simulink model "Tools"  (R2022b)
settings: Solver=ode45  StartTime=0.0  StopTime=10.0  RelTol=1e-3  EnableMultiTasking=on
undefined symbols (not defined in the file): AAopti, Copti, gam, nv_remp, Pamb, PRcrit, Rair, table_rdt_AA, Tamb, vect_delta_AA
settings Model: Creator=Boanali  LastModifiedBy=Boanali
settings DataIOCC: LimitDataPoints=on  SaveFormat=Array  SignalLoggingSaveFormat=ModelDataLogs  ReturnWorkspaceOutputs=off  SignalLoggingName=sigsOut
settings OptimizationCC: ReuseModelBlockBuffer=on
settings DebuggingCC: SaveWithParameterizedLinksMsg=none  UnderspecifiedInitializationDetection=Classic  MergeDetectMultiDrivingBlocksExec=none  SignalResolutionControl=TryResolveAllWithWarning  MultiTaskDSMMsg=warning  MultiTaskCondExecSysMsg=none  UnconnectedInputMsg=warning  UnconnectedOutputMsg=warning  UnconnectedLineMsg=warning
settings HardwareCC: ProdBitPerPointer=32  ProdBitPerSizeT=32  ProdBitPerPtrDiffT=32  ProdLargestAtomicFloat=None  ProdIntDivRoundTo=Undefined  ProdEndianess=Unspecified  ProdWordSize=32  ProdHWDeviceType=32-bit Generic  TargetUnknown=on
settings ModelReferenceCC: PropagateSignalLabelsOutOfModel=off
settings GRTTargetCC: CombineOutputUpdateFcns=off  GRTInterface=on
settings ConfigComp: CovMetricSettings=dw  CovSaveCumulativeToWorkspaceVar=on  CovSaveSingleToWorkspaceVar=on

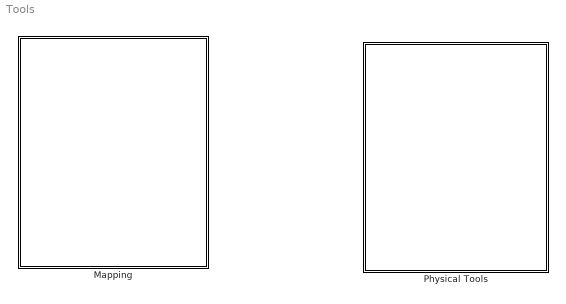
== system Tools ==
  Mapping : Subsystem
      mask Display: disp('CARTOGRAPHIES')
  Physical Tools : Subsystem
      mask Display: disp('PHYSICAL TOOLS')

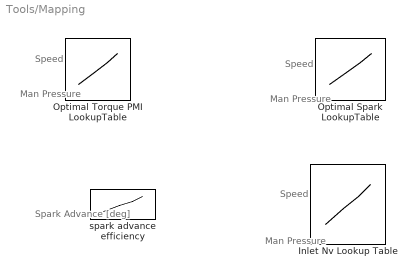
== system Tools/Mapping ==
  note: Speed
  note: Speed
  note: Spark Advance
      | [deg]
  note: Man Pressure
  note: Man Pressure
  note: Speed
  note: Man Pressure
  Inlet Nv Lookup Table : Lookup2D  RowIndex=Ne_remp  ColumnIndex=Pcol_remp  Table=nv_remp
  Optimal Spark LookupTable : Lookup2D  RowIndex=Ne_remp  ColumnIndex=Pcol_remp  Table=AAopti
  Optimal Torque PMI LookupTable : Lookup2D  RowIndex=Ne_remp  ColumnIndex=Pcol_remp  Table=Copti
  spark advance efficiency : Lookup  InputValues=vect_delta_AA  Table=table_rdt_AA

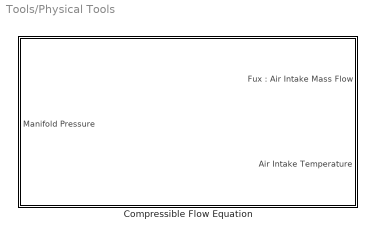
== system Tools/Physical Tools ==
  Compressible Flow Equation : Subsystem

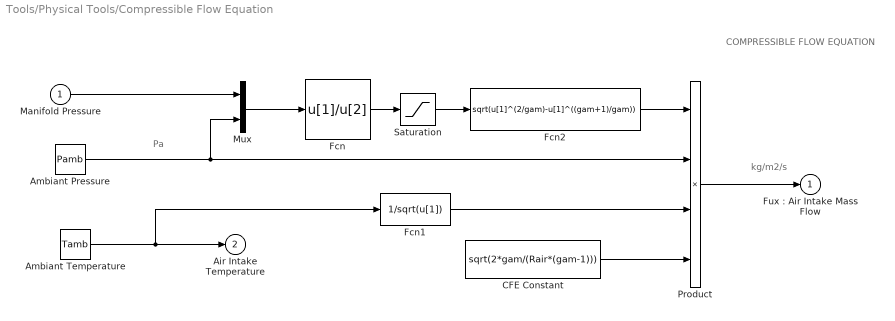
== system Tools/Physical Tools/Compressible Flow Equation ==
  note: COMPRESSIBLE FLOW EQUATION
  note: Pa
  note: kg/m2/s
  Manifold Pressure : Inport
  Ambiant Pressure : Constant  Value=Pamb
  Ambiant Temperature : Constant  Value=Tamb
  "CFE Constant " : Constant  Value=sqrt(2*gam/(Rair*(gam-1)))
  Fcn : Fcn  Expr=u[1]/u[2]
  Fcn1 : Fcn  Expr=1/sqrt(u[1])
  Fcn2 : Fcn  Expr=sqrt(u[1]^(2/gam)-u[1]^((gam+1)/gam))
  Mux : Mux  Inputs=2
  Product : Product  Inputs=4  InputSameDT=on  SaturateOnIntegerOverflow=on  OutDataTypeStr=Inherit: Same as first input
  Saturation : Saturate  UpperLimit=1  LowerLimit=PRcrit
  "Fux : Air Intake Mass Flow" : Outport
  Air Intake Temperature : Outport  Port=2
  wires:
  Ambiant Pressure/1 -> Product/2, Mux/2
  Product/1 -> "Fux : Air Intake Mass Flow"/1
  "CFE Constant "/1 -> Product/4
  Fcn2/1 -> Product/1
  Saturation/1 -> Fcn2/1
  Fcn1/1 -> Product/3
  Fcn/1 -> Saturation/1
  Mux/1 -> Fcn/1
  Manifold Pressure/1 -> Mux/1
  Ambiant Temperature/1 -> Fcn1/1, Air Intake Temperature/1
